simulink model "do178b_dhc2_rev"  (R2018b)
settings: Solver=ode23  StartTime=0.0  StopTime=25  MaxStep=1/40  RelTol=1e-2  AbsTol=1e-3  EnableMultiTasking=on
PreLoadFcn:
  | load asbdhc2_init;
  | Autopilot_bus;
model workspace (MAT data in the model file):
  ALT_Mode = [0 0 0 0 0 0 0 0 0 0 0 0 ... (1001 elements, 1001x1)]
  ALT_Ref = [991.703720962 991.703720962 991.703720962 991.703720962 991.703720962 991.703720962 991.703720962 991.703720962 991.703720962 991.703720962 991.703720962 991.703720962 ... (1001 elements, 1001x1)]
  AP_Eng = [1 1 1 1 1 1 1 1 1 1 1 1 ... (1001 elements, 1001x1)]
  AilCmdv = [0; 0; 0]
  Ail_cmd = timeseries
  Ail_cmd.Name = 'AilCmd'
  Ail_cmd.DataInfo = tsdata.datametadata
  Ail_cmd.DataInfo.Interpolation = tsdata.interpolation
  Ail_cmd.DataInfo.Interpolation.Fhandle : function handle (value not decoded)
  Ail_cmd.DataInfo.Interpolation.Name = 'zoh'
  Ail_cmd.TimeInfo = tsdata.timemetadata
  Ail_cmd.TimeInfo.Length = 1001
  Ail_cmd.TimeInfo.DuplicateTimes = 0
  Ail_cmd.TimeInfo.Increment_ = 0.025
  Ail_cmd.TimeInfo.Start_ = 0
  Ail_cmd.TimeInfo.Initialized = 1
  Ail_cmd.QualityInfo = tsdata.qualmetadata
  Ail_cmd.Data_ = [-15 -15 -15 -15 -15 -14.9375777532 -13.3004745175 -11.3988791796 -9.26136478019 -6.91375030559 -4.59638192629 -2.84726097605 ... (1001 elements, 1001x1)]
  FR = [0; 0]
  Ft = [0 0.333333333333 0.333333333333 0.333333333333 0.333333333333 0.333333333333 0.333333333333 0.333333333333 0.333333333333 0.333333333333 0.333333333333 0.333333333333 ... (1001 elements, 1001x1)]
  HDG_Mode = [0 0 0 0 0 0 0 0 0 0 0 0 ... (1001 elements, 1001x1)]
  HDG_Ref = [29.7066688805 29.7066688805 29.7066688805 29.7066688805 29.7066688805 29.7066688805 29.7066688805 29.7066688805 29.7066688805 29.7066688805 29.7066688805 29.7066688805 ... (1001 elements, 1001x1)]
  InputSize = 2
  N = 37
  PhiRefv = [0; 0; 0]
  Phi_Ref = timeseries
  Phi_Ref.DataInfo = tsdata.datametadata
  Phi_Ref.DataInfo.Interpolation = tsdata.interpolation
  Phi_Ref.DataInfo.Interpolation.Fhandle : function handle (value not decoded)
  Phi_Ref.DataInfo.Interpolation.Name = 'zoh'
  Phi_Ref.TimeInfo = tsdata.timemetadata
  Phi_Ref.TimeInfo.Length = 1001
  Phi_Ref.TimeInfo.DuplicateTimes = 0
  Phi_Ref.TimeInfo.Increment_ = 0.025
  Phi_Ref.TimeInfo.Start_ = 0
  Phi_Ref.TimeInfo.Initialized = 1
  Phi_Ref.QualityInfo = tsdata.qualmetadata
  Phi_Ref.Data_ = [-15.9132354515 -15.9132354515 -15.9132354515 -15.9132354515 -15.9132354515 -15.9132354515 -15.9132354515 -15.9132354515 -15.9132354515 -15.9132354515 -15.9132354515 -15.9132354515 ... (1001 elements, 1001x1)]
  Phiv = [0; 0; 0]
  Pwheel = [2.59796598511 2.59796598511 2.59796598511 2.59796598511 2.59796598511 2.59796598511 2.59796598511 2.59796598511 2.59796598511 2.59796598511 2.59796598511 2.59796598511 ... (1001 elements, 1001x1)]
  Roll_Mode = [1 1 1 1 1 1 1 1 1 1 1 1 ... (1001 elements, 1001x1)]
  TimeSteps = 1001
  Tkv = [0; 0; 0]
  TurnK = [-15.9132354515 -15.9132354515 -15.9132354515 -15.9132354515 -15.9132354515 -15.9132354515 -15.9132354515 -15.9132354515 -15.9132354515 -15.9132354515 -15.9132354515 -15.9132354515 ... (1001 elements, 1001x1)]
  X = [1  1  1  0  1  0  1  1  0  1  1  0  0  1  0  0  0  1  1  0  0  0  0  0  1  1  1  1  1  0  156.547682661  -34.2891675643  -6.7238554701  159.249898271  102.099492039  -128.820173923  -38.2863769545  50.7255830754  -156.969893428  -66.7656545144  -44.1886401228  34.254386326  -16.4079284241  27.0069657456  28.1914611919  -27.7076261754  -39.2522890724  9.30576559519  -30.5464722  23.1335566628  429.242036406  303.031561194  442.006699342  625.600056393  286.904020014  920.85394839  309.941229994  780.877963799  461.481818561  605.001848167  5.94264833771  -23.0798047589  -13.7340349659  0.998581267306  -11.484712041  16.7665899433  -28.6529422777  6.30898333719  24.8862140866  24.9733048405; 1  1  1  0  1  0  1  1  0  1  1  0  0  1  0  0  0  1  1  0  0  0  0  0  1  1  1  1  1  0  96.9582612885  78.4119331031  -21.1767146035  28.3602203055  77.3305381707  69.4506725412  -134.0035793  -0.896945524368  8.47338232263  127.761101236  -26.767306756  -25.3755269511  -14.0432680546  6.39760167498  -37.2438355176  11.6551504405  21.8666084099  26.859982929  21.4137725788  34.3179983117  187.482780291  320.75706466  361.884766096  938.82654512  244.599449361  926.216579676  76.4753582491  130.745166372  440.169171436  127.020527575  -22.0724594398  -3.53559927368  26.6464157318  -3.28248106537  -1.82414768299  -19.8712278416  12.5237483743  -5.17919618171  -1.36915334544  -0.185593650292]
  a = 24.9733048405
  a1 = [5.94264833771 5.94264833771 5.94264833771 5.94264833771 5.94264833771 5.94264833771 5.94264833771 5.94264833771 5.94264833771 5.94264833771 5.94264833771 5.94264833771 ... (1001 elements, 1x1001)]
  apin.time = [0 0.025 0.05 0.075 0.1 0.125 0.15 0.175 0.2 0.225 0.25 0.275 ... (1001 elements, 1001x1)]
  apin.signals(1).values = [1 1 1 1 1 1 1 1 1 1 1 1 ... (1001 elements, 1001x1)]
  apin.signals(1).dimensions = 1
  apin.signals(2).values = [0 0 0 0 0 0 0 0 0 0 0 0 ... (1001 elements, 1001x1)]
  apin.signals(2).dimensions = 1
  apin.signals(3).values = [0 0 0 0 0 0 0 0 0 0 0 0 ... (1001 elements, 1001x1)]
  apin.signals(3).dimensions = 1
  apin.signals(4).values = [156.547682661 156.547682661 156.547682661 156.547682661 156.547682661 156.547682661 156.547682661 156.547682661 156.547682661 156.547682661 156.547682661 156.547682661 ... (1001 elements, 1001x1)]
  apin.signals(4).dimensions = 1
  apin.signals(5).values = [-44.1886401228 -44.1886401228 -44.1886401228 -44.1886401228 -44.1886401228 -44.1886401228 -44.1886401228 -44.1886401228 -44.1886401228 -44.1886401228 -44.1886401228 -44.1886401228 ... (1001 elements, 1001x1)]
  apin.signals(5).dimensions = 1
  apin.signals(6).values = [429.242036406 429.242036406 429.242036406 429.242036406 429.242036406 429.242036406 429.242036406 429.242036406 429.242036406 429.242036406 429.242036406 429.242036406 ... (1001 elements, 1001x1)]
  apin.signals(6).dimensions = 1
  apin.signals(7).values = [5.94264833771 5.94264833771 5.94264833771 5.94264833771 5.94264833771 5.94264833771 5.94264833771 5.94264833771 5.94264833771 5.94264833771 5.94264833771 5.94264833771 ... (1001 elements, 1001x1)]
  apin.signals(7).dimensions = 1
  apsin.time = [0 0.025 0.05 0.075 0.1 0.125 0.15 0.175 0.2 0.225 0.25 0.275 ... (1001 elements, 1001x1)]
  curPath = '/Users/ceren.gebizli/Desktop/Shiva/QRA-Search/QRA-Search/Problems/SimulinkTesting'
  d = 71
  hws : handle (value not decoded)
  i = 11
  inertial.phi = timeseries
  inertial.phi.Name = 'phi'
  inertial.phi.DataInfo = tsdata.datametadata
  inertial.phi.DataInfo.Interpolation = tsdata.interpolation
  inertial.phi.DataInfo.Interpolation.Fhandle : function handle (value not decoded)
  inertial.phi.DataInfo.Interpolation.Name = 'zoh'
  inertial.phi.TimeInfo = tsdata.timemetadata
  inertial.phi.TimeInfo.Length = 1001
  inertial.phi.TimeInfo.DuplicateTimes = 0
  inertial.phi.TimeInfo.Increment_ = 0.025
  inertial.phi.TimeInfo.Start_ = 0
  inertial.phi.TimeInfo.Initialized = 1
  inertial.phi.QualityInfo = tsdata.qualmetadata
  inertial.phi.Data_ = [-8.01936314143e-16 0.000181471818699 -0.00121043131907 -0.00754243025641 -0.0220135457189 -0.0474649089937 -0.086409509468 -0.141054755662 -0.213300660829 -0.304830987454 -0.416623623067 -0.545698165105 ... (1001 elements, 1001x1)]
  inertial.theta = timeseries
  inertial.theta.Name = 'theta'
  inertial.theta.DataInfo = tsdata.datametadata
  inertial.theta.DataInfo.Interpolation = tsdata.interpolation
  inertial.theta.DataInfo.Interpolation.Fhandle : function handle (value not decoded)
  inertial.theta.DataInfo.Interpolation.Name = 'zoh'
  inertial.theta.TimeInfo = tsdata.timemetadata
  inertial.theta.TimeInfo.Length = 1001
  inertial.theta.TimeInfo.DuplicateTimes = 0
  inertial.theta.TimeInfo.Increment_ = 0.025
  inertial.theta.TimeInfo.Start_ = 0
  inertial.theta.TimeInfo.Initialized = 1
  inertial.theta.QualityInfo = tsdata.qualmetadata
  inertial.theta.Data_ = [7.46541826999 7.46398070067 7.45666172375 7.43805804315 7.40283654619 7.34702482868 7.27332345058 7.18849824115 7.09958585144 7.01321197914 6.93468614303 6.86454921985 ... (1001 elements, 1001x1)]
  inertial.psi = timeseries
  inertial.psi.Name = 'psi'
  inertial.psi.DataInfo = tsdata.datametadata
  inertial.psi.DataInfo.Interpolation = tsdata.interpolation
  inertial.psi.DataInfo.Interpolation.Fhandle : function handle (value not decoded)
  inertial.psi.DataInfo.Interpolation.Name = 'zoh'
  inertial.psi.TimeInfo = tsdata.timemetadata
  inertial.psi.TimeInfo.Length = 1001
  inertial.psi.TimeInfo.DuplicateTimes = 0
  inertial.psi.TimeInfo.Increment_ = 0.025
  inertial.psi.TimeInfo.Start_ = 0
  inertial.psi.TimeInfo.Initialized = 1
  inertial.psi.QualityInfo = tsdata.qualmetadata
  inertial.psi.Data_ = [113 112.999723859 112.998881527 112.997491019 112.995622363 112.993388908 112.990947692 112.988509003 112.986332158 112.984697602 112.98390006 112.984240621 ... (1001 elements, 1001x1)]
  inertial.p = timeseries
  inertial.p.Name = 'p'
  inertial.p.DataInfo = tsdata.datametadata
  inertial.p.DataInfo.Interpolation = tsdata.interpolation
  inertial.p.DataInfo.Interpolation.Fhandle : function handle (value not decoded)
  inertial.p.DataInfo.Interpolation.Name = 'zoh'
  inertial.p.TimeInfo = tsdata.timemetadata
  inertial.p.TimeInfo.Length = 1001
  inertial.p.TimeInfo.DuplicateTimes = 0
  inertial.p.TimeInfo.Increment_ = 0.025
  inertial.p.TimeInfo.Start_ = 0
  inertial.p.TimeInfo.Initialized = 1
  inertial.p.QualityInfo = tsdata.qualmetadata
  inertial.p.Data_ = [0 0.000348389974139 -0.126229012603 -0.387182020206 -0.769798889218 -1.26011690282 -1.8453170072 -2.51380447813 -3.25536090727 -4.06077105791 -4.84938742553 -5.44201618039 ... (1001 elements, 1001x1)]
  inertial.q = timeseries
  inertial.q.Name = 'q'
  inertial.q.DataInfo = tsdata.datametadata
  inertial.q.DataInfo.Interpolation = tsdata.interpolation
  inertial.q.DataInfo.Interpolation.Fhandle : function handle (value not decoded)
  inertial.q.DataInfo.Interpolation.Name = 'zoh'
  inertial.q.TimeInfo = tsdata.timemetadata
  inertial.q.TimeInfo.Length = 1001
  inertial.q.TimeInfo.DuplicateTimes = 0
  inertial.q.TimeInfo.Increment_ = 0.025
  inertial.q.TimeInfo.Start_ = 0
  inertial.q.TimeInfo.Initialized = 1
  inertial.q.QualityInfo = tsdata.qualmetadata
  inertial.q.Data_ = [0 -0.141109022992 -0.481834459904 -1.04195937266 -1.80804605852 -2.62895783334 -3.21861628739 -3.52029801203 -3.54830041644 -3.3203997107 -2.96034825264 -2.67963325159 ... (1001 elements, 1001x1)]
  inertial.r = timeseries
  inertial.r.Name = 'r'
  inertial.r.DataInfo = tsdata.datametadata
  inertial.r.DataInfo.Interpolation = tsdata.interpolation
  inertial.r.DataInfo.Interpolation.Fhandle : function handle (value not decoded)
  inertial.r.DataInfo.Interpolation.Name = 'zoh'
  inertial.r.TimeInfo = tsdata.timemetadata
  inertial.r.TimeInfo.Length = 1001
  inertial.r.TimeInfo.DuplicateTimes = 0
  inertial.r.TimeInfo.Increment_ = 0.025
  inertial.r.TimeInfo.Start_ = 0
  inertial.r.TimeInfo.Initialized = 1
  inertial.r.QualityInfo = tsdata.qualmetadata
  inertial.r.Data_ = [0 -0.0220962935685 -0.0445610325511 -0.0653499435324 -0.0828788100931 -0.0961239290518 -0.103184615316 -0.102017006398 -0.0907675753211 -0.0679797938768 -0.0324798838026 0.0140525471681 ... (1001 elements, 1001x1)]
  j = 7
  list(1).name = 'ALT_Mode'
  list(1).size = [1001 1]
  list(1).bytes = 8008
  list(1).class = 'double'
  list(1).global = 0
  list(1).sparse = 0
  list(1).complex = 0
  list(1).nesting.function = 'simroll_ap'
  list(1).nesting.level = 1
  list(1).persistent = 0
  list(2).name = 'ALT_Ref'
  list(2).size = [1001 1]
  list(2).bytes = 8008
  list(2).class = 'double'
  list(2).global = 0
  list(2).sparse = 0
  list(2).complex = 0
  list(2).nesting.function = 'simroll_ap'
  list(2).nesting.level = 1
  list(2).persistent = 0
  list(3).name = 'AP_Eng'
  list(3).size = [1001 1]
  list(3).bytes = 8008
  list(3).class = 'double'
  list(3).global = 0
  list(3).sparse = 0
  list(3).complex = 0
  list(3).nesting.function = 'simroll_ap'
  list(3).nesting.level = 1
  list(3).persistent = 0
  list(4).name = 'AilCmdv'
  list(4).size = [3 1]
  list(4).bytes = 24
  list(4).class = 'double'
  list(4).global = 0
  list(4).sparse = 0
  list(4).complex = 0
  list(4).nesting.function = 'simroll_ap'
  list(4).nesting.level = 1
  list(4).persistent = 0
  list(5).name = 'Ail_cmd'
  list(5).size = [1 1]
  list(5).bytes = 8892
  list(5).class = 'timeseries'
  list(5).global = 0
  list(5).sparse = 0
  list(5).complex = 0
  list(5).nesting.function = 'simroll_ap'
  list(5).nesting.level = 1
  list(5).persistent = 0
  list(6).name = 'FR'
  list(6).size = [2 1]
  list(6).bytes = 16
  list(6).class = 'double'
  list(6).global = 0
  list(6).sparse = 0
  list(6).complex = 0
  list(6).nesting.function = 'simroll_ap'
  list(6).nesting.level = 1
  list(6).persistent = 0
  list(7).name = 'Ft'
  list(7).size = [1001 1]
  list(7).bytes = 8008
  list(7).class = 'double'
  list(7).global = 0
  list(7).sparse = 0
  list(7).complex = 0
  list(7).nesting.function = 'simroll_ap'
  list(7).nesting.level = 1
  list(7).persistent = 0
  list(8).name = 'HDG_Mode'
  list(8).size = [1001 1]
  list(8).bytes = 8008
  list(8).class = 'double'
  list(8).global = 0
  list(8).sparse = 0
  list(8).complex = 0
  list(8).nesting.function = 'simroll_ap'
  list(8).nesting.level = 1
  list(8).persistent = 0
  list(9).name = 'HDG_Ref'
  list(9).size = [1001 1]
  list(9).bytes = 8008
  list(9).class = 'double'
  list(9).global = 0
  list(9).sparse = 0
  list(9).complex = 0
  list(9).nesting.function = 'simroll_ap'
  list(9).nesting.level = 1
  list(9).persistent = 0
  list(10).name = 'InputSize'
  list(10).size = [1 1]
  list(10).bytes = 8
  list(10).class = 'double'
  list(10).global = 0
  list(10).sparse = 0
  list(10).complex = 0
  list(10).nesting.function = 'simroll_ap'
  list(10).nesting.level = 1
  list(10).persistent = 0
  list(11).name = 'N'
  list(11).size = [1 1]
  list(11).bytes = 8
  list(11).class = 'double'
  list(11).global = 0
  list(11).sparse = 0
  list(11).complex = 0
  list(11).nesting.function = 'simroll_ap'
  list(11).nesting.level = 1
  list(11).persistent = 0
  list(12).name = 'PhiRefv'
  list(12).size = [3 1]
  list(12).bytes = 24
  list(12).class = 'double'
  list(12).global = 0
  list(12).sparse = 0
  list(12).complex = 0
  list(12).nesting.function = 'simroll_ap'
  list(12).nesting.level = 1
  list(12).persistent = 0
  list(13).name = 'Phi_Ref'
  list(13).size = [1 1]
  list(13).bytes = 8880
  list(13).class = 'timeseries'
  list(13).global = 0
  list(13).sparse = 0
  list(13).complex = 0
  list(13).nesting.function = 'simroll_ap'
  list(13).nesting.level = 1
  list(13).persistent = 0
  list(14).name = 'Phiv'
  list(14).size = [3 1]
  list(14).bytes = 24
  list(14).class = 'double'
  list(14).global = 0
  list(14).sparse = 0
  list(14).complex = 0
  list(14).nesting.function = 'simroll_ap'
  list(14).nesting.level = 1
  list(14).persistent = 0
  list(15).name = 'Pwheel'
  list(15).size = [1001 1]
  list(15).bytes = 8008
  list(15).class = 'double'
  list(15).global = 0
  list(15).sparse = 0
  list(15).complex = 0
  list(15).nesting.function = 'simroll_ap'
  list(15).nesting.level = 1
  list(15).persistent = 0
  list(16).name = 'Roll_Mode'
  list(16).size = [1001 1]
  list(16).bytes = 8008
  list(16).class = 'double'
  list(16).global = 0
  list(16).sparse = 0
  list(16).complex = 0
  list(16).nesting.function = 'simroll_ap'
  list(16).nesting.level = 1
  list(16).persistent = 0
  list(17).name = 'TimeSteps'
  list(17).size = [1 1]
  list(17).bytes = 8
  list(17).class = 'double'
  list(17).global = 0
  list(17).sparse = 0
  list(17).complex = 0
  list(17).nesting.function = 'simroll_ap'
  list(17).nesting.level = 1
  list(17).persistent = 0
  list(18).name = 'Tkv'
  list(18).size = [3 1]
  list(18).bytes = 24
  list(18).class = 'double'
  list(18).global = 0
  list(18).sparse = 0
  list(18).complex = 0
  list(18).nesting.function = 'simroll_ap'
  list(18).nesting.level = 1
  list(18).persistent = 0
  list(19).name = 'TurnK'
  list(19).size = [1001 1]
  list(19).bytes = 8008
  list(19).class = 'double'
  list(19).global = 0
  list(19).sparse = 0
  list(19).complex = 0
  list(19).nesting.function = 'simroll_ap'
  list(19).nesting.level = 1
  list(19).persistent = 0
  list(20).name = 'X'
  list(20).size = [2 70]
  list(20).bytes = 1120
  list(20).class = 'double'
  list(20).global = 0
  list(20).sparse = 0
  list(20).complex = 0
  list(20).nesting.function = 'simroll_ap'
  list(20).nesting.level = 1
  list(20).persistent = 0
  list(21).name = 'a'
  list(21).size = [1 1]
  list(21).bytes = 8
  list(21).class = 'double'
  list(21).global = 0
  list(21).sparse = 0
  list(21).complex = 0
  list(21).nesting.function = 'simroll_ap'
  list(21).nesting.level = 1
  list(21).persistent = 0
  list(22).name = 'a1'
  list(22).size = [1 1001]
  list(22).bytes = 8008
  list(22).class = 'double'
  list(22).global = 0
  list(22).sparse = 0
  list(22).complex = 0
  list(22).nesting.function = 'simroll_ap'
  list(22).nesting.level = 1
  list(22).persistent = 0
  list(23).name = 'apin'
  list(23).size = [1 1]
  list(23).bytes = 66168
  list(23).class = 'struct'
  list(23).global = 0
  list(23).sparse = 0
  list(23).complex = 0
  list(23).nesting.function = 'simroll_ap'
  list(23).nesting.level = 1
  list(23).persistent = 0
  list(24).name = 'curPath'
  list(24).size = [1 81]
  list(24).bytes = 162
  list(24).class = 'char'
  list(24).global = 0
  list(24).sparse = 0
  list(24).complex = 0
  list(24).nesting.function = 'simroll_ap'
  list(24).nesting.level = 1
  list(24).persistent = 0
  list(25).name = 'd'
  list(25).size = [1 1]
  list(25).bytes = 8
  list(25).class = 'double'
  list(25).global = 0
  list(25).sparse = 0
  list(25).complex = 0
  list(25).nesting.function = 'simroll_ap'
  list(25).nesting.level = 1
  list(25).persistent = 0
  list(26).name = 'hws'
  list(26).size = [1 1]
  list(26).bytes = 0
  list(26).class = 'Simulink.ModelWorkspace'
  list(26).global = 0
  list(26).sparse = 0
  list(26).complex = 0
  list(26).nesting.function = 'simroll_ap'
  list(26).nesting.level = 1
  list(26).persistent = 0
  list(27).name = 'i'
  list(27).size = [1 1]
  list(27).bytes = 8
  list(27).class = 'double'
  list(27).global = 0
  list(27).sparse = 0
  list(27).complex = 0
  list(27).nesting.function = 'simroll_ap'
  list(27).nesting.level = 1
  list(27).persistent = 0
  list(28).name = 'inertial'
  list(28).size = [1 1]
  list(28).bytes = 54364
  list(28).class = 'struct'
  list(28).global = 0
  list(28).sparse = 0
  list(28).complex = 0
  list(28).nesting.function = 'simroll_ap'
  list(28).nesting.level = 1
  list(28).persistent = 0
  list(29).name = 'j'
  list(29).size = [1 1]
  list(29).bytes = 8
  list(29).class = 'double'
  list(29).global = 0
  list(29).sparse = 0
  list(29).complex = 0
  list(29).nesting.function = 'simroll_ap'
  list(29).nesting.level = 1
  list(29).persistent = 0
  list(30).name = 'list'
  list(30).size = [17 1]
  list(30).bytes = 25008
  list(30).class = 'struct'
  list(30).global = 0
  list(30).sparse = 0
  list(30).complex = 0
  list(30).nesting.function = 'simroll_ap'
  list(30).nesting.level = 1
  list(30).persistent = 0
  list(31).name = 'modelpath'
  list(31).size = [1 108]
  list(31).bytes = 216
  list(31).class = 'char'
  list(31).global = 0
  list(31).sparse = 0
  list(31).complex = 0
  list(31).nesting.function = 'simroll_ap'
  list(31).nesting.level = 1
  list(31).persistent = 0
  list(32).name = 'models'
  list(32).size = [1 9]
  list(32).bytes = 3286
  list(32).class = 'cell'
  list(32).global = 0
  list(32).sparse = 0
  list(32).complex = 0
  list(32).nesting.function = 'simroll_ap'
  list(32).nesting.level = 1
  list(32).persistent = 0
  list(33).name = 'n'
  list(33).size = [1 1]
  list(33).bytes = 8
  list(33).class = 'double'
  list(33).global = 0
  list(33).sparse = 0
  list(33).complex = 0
  list(33).nesting.function = 'simroll_ap'
  list(33).nesting.level = 1
  list(33).persistent = 0
  list(34).name = 'nbrInputs'
  list(34).size = [1 1]
  list(34).bytes = 8
  list(34).class = 'double'
  list(34).global = 0
  list(34).sparse = 0
  list(34).complex = 0
  list(34).nesting.function = 'simroll_ap'
  list(34).nesting.level = 1
  list(34).persistent = 0
  list(35).name = 'rollOut'
  list(35).size = [0 0]
  list(35).bytes = 0
  list(35).class = 'double'
  list(35).global = 0
  list(35).sparse = 0
  list(35).complex = 0
  list(35).nesting.function = 'simroll_ap'
  list(35).nesting.level = 1
  list(35).persistent = 0
  list(36).name = 'simOut'
  list(36).size = [1 1]
  list(36).bytes = 225127
  list(36).class = 'Simulink.SimulationOutput'
  list(36).global = 0
  list(36).sparse = 0
  list(36).complex = 0
  list(36).nesting.function = 'simroll_ap'
  list(36).nesting.level = 1
  list(36).persistent = 0
  list(37).name = 't'
  list(37).size = [1 1]
  list(37).bytes = 8
  list(37).class = 'double'
  list(37).global = 0
  list(37).sparse = 0
  list(37).complex = 0
  list(37).nesting.function = 'simroll_ap'
  list(37).nesting.level = 1
  list(37).persistent = 0
  modelpath = '/Users/ceren.gebizli/Desktop/Shiva/QRA-Search/QRA-Search/SimulinkModels/autopilot_R2013b_workarea/aprevised/'
  models = {'/Users/ceren.gebizli/Desktop/Shiva/QRA-Search/QRA-Search/SimulinkModels/autopilot_R2013b_workarea/aprevised/roll_ap_rev.slx', '/Users/ceren.gebizli/Desktop/Shiva/QRA-Search/QRA-Search/SimulinkModels/autopilot_R2013b_workarea/aprevised/yaw_damper_rev.slx', '/Users/ceren.gebizli/Desktop/Shiva/QRA-Search/QRA-Search/SimulinkModels/autopilot_R2013b_workarea/aprevised/pitch_ap_rev.slx', '/Users/ceren.gebizli/Desktop/Shiva/QRA-Search/QRA-Search/SimulinkModels/autopilot_R2013b_workarea/aprevised/Autopilot_rev.slx', '/Users/ceren.gebizli/Desktop/Shiva/QRA-Search/QRA-Search/SimulinkModels/autopilot_R2013b_workarea/aprevised/AP_Lib_rev.slx', '/Users/ceren.gebizli/Desktop/Shiva/QRA-Search/QRA-Search/SimulinkModels/autopilot_R2013b_workarea/aprevised/Heading_Mode_rev.slx', '/Users/ceren.gebizli/Desktop/Shiva/QRA-Search/QRA-Search/SimulinkModels/autopilot_R2013b_workarea/aprevised/attitude_controller_rev.slx', '/Users/ceren.gebizli/Desktop/Shiva/QRA-Search/QRA-Search/SimulinkModels/autopilot_R2013b_workarea/aprevised/Altitude_Mode_rev.slx', '/Users/ceren.gebizli/Desktop/Shiva/QRA-Search/QRA-Search/SimulinkModels/autopilot_R2013b_workarea/aprevised/do178b_dhc2_rev.slx'}
  n = 1
  nbrInputs = 7
  rollOut = []
  simOut : Simulink.SimulationOutput (value not decoded)
  t = [0 0.025 0.05 0.075 0.1 0.125 0.15 0.175 0.2 0.225 0.25 0.275 ... (1001 elements, 1x1001)]
undefined symbols (not defined in the file): beaver_b, beaver_c, beaver_init_p, beaver_init_pitch, beaver_init_q, beaver_init_r, beaver_init_roll, beaver_mass, Cl0, Cl_alpha2_dpt, Cl_beta, Cl_da, Cl_da_alpha, Cl_dr, Cl_p, Cl_r, Cm0, Cm_alpha, Cm_alpha2, Cm_beta2, Cm_de, Cm_df, Cm_dpt, Cm_q, Cm_r, Cn0, Cn_beta, Cn_beta3, Cn_da, Cn_dpt3, Cn_dr, Cn_p, Cn_q, Cn_r, Cx0, Cx_alpha, Cx_alpha2, Cx_alpha3, Cx_df, Cx_df_alpha, Cx_dpt, Cx_dpt2_alpha, Cx_dr, Cx_q, Cy0, Cy_beta, Cy_da, Cy_dr, Cy_dr_alpha, Cy_p, Cy_r, Cz0, Cz_alpha, Cz_alpha3, Cz_de, Cz_de_beta, Cz_df, Cz_df_alpha, Cz_dpt, Cz_q ... (+9)
libraries: aerolibconvert2 x6, simulink x6, aerolibobsolete x5, aerolibasang x3, aerolibwind2 x3, aerolibadyn x1, aerolibatmos2 x1
(part 1 of 3)
Description:
  | Fly the DeHavilland Beaver
  | 
  | This demonstration uses a pilot's joystick to allow you to fly the DeHavilland
  | Beaver modeled with Simulnk, and Aerospace Blockset.  This model has been
  | color coded to aid in locating Aerospace Blockset blocks. The red blocks are
  | Aerospace Blockset blocks, the orange blocks are subsystems containing
  | additional Aerospace Blockset blocks and the white blocks are Simulink blocks.
  | 
  | The DeHavilland Beaver model includes the airframe dynamics, including
  | aerodynamics. Effects of the environment are also modeled, such as wind profiles
  | for the landing phase. Visualization for this model is done via an interface to
  | FlightGear, a open source flight simulator package.
  | 
  | The DeHavilland Beaver was first flown in 1947. Today it is still prized by pilots
  | for its reliability and versatility. The DeHavilland Beaver can be operated on wheels,
  | skis or float landing gear.
  | 
  | Speed Max       110 kts
  | Altitude Max 10,000 ft
  | Range Max       400 nm
  | Load                     6 passengers
  | Crew                     1 member
  | 
  | For more information on the FlightGear interface, see the documentation.
settings Model: ExtModeTrigMode=oneshot  ExtModeArmWhenConnect=off  ExtModeAutoUpdateStatusClock=off  Creator=The MathWorks Inc.  LastModifiedBy=khouloud.gaaloul
settings SolverCC: AutoScaleAbsTol=off
settings DataIOCC: ExternalInput=apin  LoadExternalInput=on  SaveFormat=Array  SaveOutput=off  DSMLogging=off  SaveTime=off  SignalLoggingName=sigsOut
settings OptimizationCC: BlockReduction=off  ConditionallyExecuteInputs=off  ExpressionDepthLimit=2147483647  InitFltsAndDblsToZero=on  EfficientFloat2IntCast=on  LifeSpan=inf
settings DebuggingCC: SignalInfNanChecking=error  ReadBeforeWriteMsg=EnableAllAsError  WriteAfterWriteMsg=EnableAllAsError  WriteAfterReadMsg=EnableAllAsError  AlgebraicLoopMsg=error  ArtificialAlgebraicLoopMsg=error  SaveWithParameterizedLinksMsg=none  UnderspecifiedInitializationDetection=Classic  MergeDetectMultiDrivingBlocksExec=none  CheckExecutionContextPreStartOutputMsg=on  CheckExecutionContextRuntimeOutputMsg=on  BlockPriorityViolationMsg=error  MaxConsecutiveZCsMsg=warning  SolverPrmCheckMsg=warning  InheritedTsInSrcMsg=error  SigSpecEnsureSampleTimeMsg=error  CheckMatrixSingularityMsg=error  IntegerOverflowMsg=error  ParameterUnderflowMsg=error  ParameterPrecisionLossMsg=error  UnnecessaryDatatypeConvMsg=warning  VectorMatrixConversionMsg=warning  FcnCallInpInsideContextMsg=warning  SignalLabelMismatchMsg=warning  UnconnectedInputMsg=error  UnconnectedOutputMsg=error  UnconnectedLineMsg=error  SFcnCompatibilityMsg=warning  BusObjectLabelMismatch=error  RootOutportRequireBusObject=error  AssertControl=DisableAll  ModelReferenceIOMsg=error  ModelReferenceIOMismatchMessage=error  UnknownTsInhSupMsg=error  ModelReferenceDataLoggingMessage=error  StateNameClashWarn=warning  SFUnexpectedBacktrackingDiag=warning  SFNoUnconditionalDefaultTransitionDiag=warning  SFExecutionAtInitializationDiag=none  IntegerSaturationMsg=error
settings HardwareCC: ProdBitPerPointer=32  ProdBitPerSizeT=32  ProdBitPerPtrDiffT=32  ProdLargestAtomicFloat=None  ProdEndianess=BigEndian  ProdWordSize=32  ProdHWDeviceType=32-bit Embedded Processor  TargetHWDeviceType=32-bit Generic  ProdEqTarget=off
settings ModelReferenceCC: CheckModelReferenceTargetMessage=none  PropagateSignalLabelsOutOfModel=off
settings SFSimCC: SimUseLocalCustomCode=off  MATLABDynamicMemAlloc=off
settings RTWCC: SystemTargetFile=ert.tlc  TemplateMakefile=ert_default_tmf  Description=Real-Time Workshop Embedded Coder (no auto configuration)  RTWVerbose=off  RTWUseLocalCustomCode=off
settings CodeAppCC: ForceParamTrailComments=on  IgnoreCustomStorageClasses=off  MangleLength=4  CustomSymbolStrType=$N$R$M  StateflowObjectComments=on  InternalIdentifier=Classic  ReqsInCode=on
settings ERTTargetCC: TargetFcnLib=ansi_tfl_tmw.mat  MultiwordLength=2048  GenerateSampleERTMain=on  IncludeMdlTerminateFcn=off  SuppressErrorStatus=on  SupportAbsoluteTime=off  SupportNonFinite=off  SupportComplex=off  ERTCustomFileTemplate=example_file_process.tlc  ConvertIfToSwitch=off  SuppressUnreachableDefaultCases=off
settings ConfigComp: CovScope=ReferencedModels  CovIncludeTopModel=off  CovMetricSettings=dcmtrzoiwe  CovHTMLOptions=-sRT=1 -aTS=1 -bRG=1 -bTC=1 -hTR=0 -nFC=0 -scm=1 -bcm=1 -xEv=0  CovSaveCumulativeToWorkspaceVar=on  CovCumulativeReport=on  CovShowResultsExplorer=off  CovReportOnPause=off  CovExternalEMLEnable=off

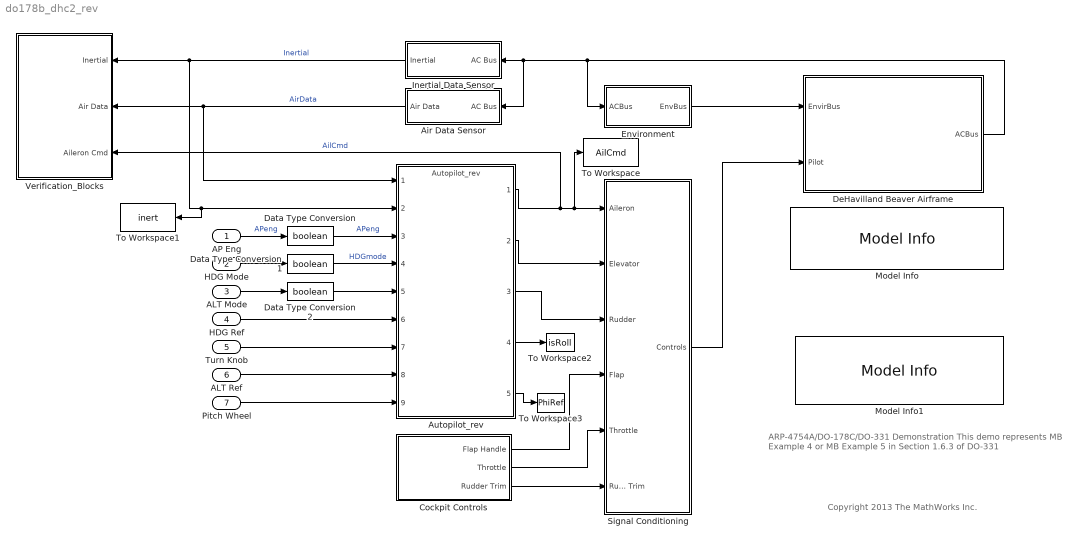
== system do178b_dhc2_rev ==
  note: Copyright 2013 The MathWorks Inc.
  note: ARP-4754A/DO-178C/DO-331 Demonstration
      | This demo represents MB Example 4 or
      | MB Example 5 in Section 1.6.3 of DO-331
  AP Eng : Inport  OutMin=0  OutMax=1  OutDataTypeStr=double  PortDimensions=1  SampleTime=[0.025000000000000001,0]
  HDG Mode : Inport  Port=2  OutMin=0  OutMax=1  OutDataTypeStr=double  PortDimensions=1  SampleTime=[0.025000000000000001,0]
  ALT Mode : Inport  Port=3  OutMin=0  OutMax=1  OutDataTypeStr=double  PortDimensions=1  SampleTime=[0.025000000000000001,0]
  HDG Ref : Inport  Port=4  OutMin=-180  OutMax=180  OutDataTypeStr=double  PortDimensions=1  SampleTime=[0.025000000000000001,0]
  Turn Knob : Inport  Port=5  OutMin=-45  OutMax=45  OutDataTypeStr=double  PortDimensions=1  SampleTime=[0.025000000000000001,0]
  ALT Ref : Inport  Port=6  OutMin=0  OutMax=65000  OutDataTypeStr=double  PortDimensions=1  SampleTime=[0.025000000000000001,0]
  Pitch Wheel : Inport  Port=7  OutMin=-30  OutMax=30  OutDataTypeStr=double  PortDimensions=1  SampleTime=[0.025000000000000001,0]
  Air Data Sensor : Subsystem  TreatAsAtomicUnit=on
  Autopilot_rev : ModelReference  ModelNameDialog=Autopilot_rev  SimulationMode=Normal  ModelReferenceVersion=1.171
  Cockpit Controls : Subsystem  Tag=STV Subsys  LoadFcn=sigbuilder_block('load');  StartFcn=sigbuilder_block('start');  StopFcn=sigbuilder_block('stop');  ClipboardFcn=sigbuilder_block('clipboard');  mask(Sigbuilder block){tuvar=[0:10]}
      mask help: Sigbuilder GUI
      mask init:
      | if ~strcmp(get_param(bdroot(gcbh),'SimulationStatus'),'stopped') tuvar = sigbuilder_block('maskInit'); end
      settings: CopyFcn=sigbuilder_block('copy');  DeleteFcn=sigbuilder_block('delete');  ModelCloseFcn=sigbuilder_block('modelClose');  PreSaveFcn=sigbuilder_block('preSave');  PauseFcn=sigbuilder_block('pause')  ContinueFcn=sigbuilder_block('continue')  NameChangeFcn=sigbuilder_block('namechange');  OpenFcn=sigbuilder_block('open',[144.75 92.25 575.25 393 ]);  CloseFcn=sigbuilder_block('close');
      mask Display: plot(0, 0, 100, 100,[2, 2, 32, 32, 2], [68, 8, 8, 68, 68],[32, 2], [38, 38], [32, 19, 2],[53, 60, 44], [32, 17, 17, 2],[16, 16, 31, 31]);txt = getActiveGroup(gcbh);text(2, 100, txt,'verticalAlignment', 'top');
  Data Type Conversion : DataTypeConversion  OutDataTypeStr=boolean
  Data Type Conversion1 : DataTypeConversion  OutDataTypeStr=boolean
  Data Type Conversion2 : DataTypeConversion  OutDataTypeStr=boolean
  DeHavilland Beaver Airframe : Subsystem
      mask Display: image(imread('asbbeaver.jpg'))
  Environment : Subsystem
  Inertial Data Sensor : Subsystem  TreatAsAtomicUnit=on
  Model Info : simulink/Model-Wide Utilities/Model Info  Frame=on  DisplayStringWithTags=|  HorizontalTextAlignment=Center  LeftAlignmentValue=0.5
      | DeHavilland Beaver model 
      | based on original work created by
      | Marc Rauw for Delft University of Technology.  
      | http://www.dutchroll.com
  Model Info1 : simulink/Model-Wide Utilities/Model Info  Frame=on  DisplayStringWithTags=|  HorizontalTextAlignment=Left  LeftAlignmentValue=0.02
      | ARP-4754A/DO-178C/DO-331 Demonstration
      | Author: %<LastModifiedBy>
      | Model Version: %<ModelVersion>
      | Date: %<LastModificationDate>
  Signal Conditioning : Subsystem
  To Workspace : ToWorkspace  VariableName=AilCmd  SaveFormat=Timeseries  SampleTime=-1
  To Workspace1 : ToWorkspace  VariableName=inert  SaveFormat=Timeseries  SampleTime=-1
  To Workspace2 : ToWorkspace  VariableName=isRoll  SaveFormat=Timeseries  SampleTime=-1
  To Workspace3 : ToWorkspace  VariableName=PhiRef  SaveFormat=Timeseries  SampleTime=-1
  Verification_Blocks : Subsystem
  wires:
  DeHavilland Beaver Airframe/1(ACBus) -> Inertial Data Sensor/1(AC Bus), Air Data Sensor/1(AC Bus), Environment/1(ACBus)
  Environment/1(EnvBus) -> DeHavilland Beaver Airframe/1(EnvirBus)
  Signal Conditioning/1(Controls) -> DeHavilland Beaver Airframe/2(Pilot)
  Autopilot_rev/1 -> To Workspace/1, Signal Conditioning/1(Aileron), Verification_Blocks/3(Aileron Cmd)  "AilCmd"
  Air Data Sensor/1(Air Data) -> Autopilot_rev/1, Verification_Blocks/2(Air Data)  "AirData"
  Inertial Data Sensor/1(Inertial) -> To Workspace1/1, Autopilot_rev/2, Verification_Blocks/1(Inertial)  "Inertial"
  Autopilot_rev/2 -> Signal Conditioning/2(Elevator)
  Autopilot_rev/3 -> Signal Conditioning/3(Rudder)
  Cockpit Controls/1(Flap Handle) -> Signal Conditioning/4(Flap)
  Cockpit Controls/2(Throttle) -> Signal Conditioning/5(Throttle)
  Cockpit Controls/3(Rudder Trim) -> Signal Conditioning/6(Rudder Trim)
  Data Type Conversion/1 -> Autopilot_rev/3  "APeng"
  Data Type Conversion1/1 -> Autopilot_rev/4  "HDGmode"
  Data Type Conversion2/1 -> Autopilot_rev/5
  AP Eng/1 -> Data Type Conversion/1  "APeng"
  HDG Mode/1 -> Data Type Conversion1/1
  ALT Mode/1 -> Data Type Conversion2/1
  HDG Ref/1 -> Autopilot_rev/6
  Turn Knob/1 -> Autopilot_rev/7
  ALT Ref/1 -> Autopilot_rev/8
  Pitch Wheel/1 -> Autopilot_rev/9
  Autopilot_rev/4 -> To Workspace2/1
  Autopilot_rev/5 -> To Workspace3/1
